simulink model "testing_C_functions5"  (R2020b)
settings: Solver=VariableStepAuto  StartTime=0.0  StopTime=1.5  FixedStep=Ts
undefined symbols (not defined in the file or in its folder): A_frq_step, A_phase_step, DiscIntNeverNeededParam, f_rad, k_phi, ki, kp, N, t_frq_step, t_phase_step, Ts, V_g, var_noise
libraries: simulink x10, bach_library x6
settings Model: Creator=Kasper Laustsen  LastModifiedBy=Kasper Laustsen
settings DataIOCC: ExternalInput=tt1  LoadExternalInput=on
settings SFSimCC: SimCustomHeaderCode=|
  | #include "PLL.h"
  | #include "MAF.h"
settings SFSimCC: SimUserSources=|
  | PLL.c
  | MAF.c

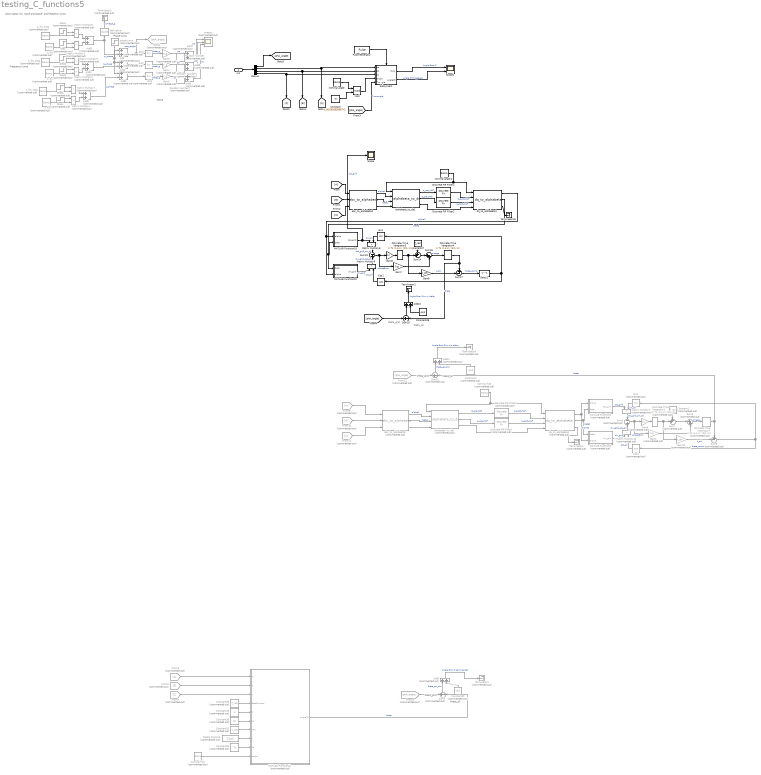
== system testing_C_functions5 ==
  note: Noise
  note: Phase-jump
  note: Input signal incl. noise and phase- and frequency jump
  note: Frequency-jump
  note: theta_pll
  note: theta_grid
  note: theta_pll
  note: theta_grid
  note: theta_pll
  note: theta_grid
  In1 : Inport
  Add{,1..9,11} (11 alike) : Sum  Commented=on
  Add10 : Sum
  Constant : Constant  Value=3.1415926535897*2
  Constant1 : Constant  Commented=on  Value=f_rad
  Constant2 : Constant  Commented=on  Value=-pi/2
  Constant25 : Constant  Commented=on  Value=Ts
  Constant26 : Constant  Commented=on  Value=f_rad
  Constant27 : Constant  Value=f_rad
  Constant28 : Constant  Value=-pi/2
  Constant29 : Constant  Commented=on  Value=ki
  Constant30 : Constant  Commented=on  Value=kp
  Constant31 : Constant  Commented=on  Value=k_phi
  Constant32 : Constant  Commented=on  Value=-pi/2
  Cos1 : Trigonometry  Operator=cos
  Cos2 : Trigonometry  Commented=on  Operator=cos
  Delay2 : Delay  DelayLength=1
  Demux : Demux
  Derivative : Derivative  Commented=on
  Digital Clock12 : DigitalClock  Commented=on  SampleTime=Ts
  Discrete FIR Filter1 : DiscreteFir  Commented=on  Coefficients=[ones(1,round(N)).*1/N]  SampleTime=Ts
  Discrete FIR Filter2 : DiscreteFir  Coefficients=[ones(1,round(N)).*1/N]  SampleTime=Ts
  Discrete FIR Filter3 : DiscreteFir  Commented=on  Coefficients=[ones(1,round(N)).*1/N]  SampleTime=Ts
  Discrete FIR Filter4 : DiscreteFir  Coefficients=[ones(1,round(N)).*1/N]  SampleTime=Ts
  Discrete-Time Integrator1 : DiscreteIntegrator  Commented=on  IntegratorMethod=Integration: Trapezoidal  SampleTime=-1  ICPrevOutput=DiscIntNeverNeededParam  ICPrevScaledInput=DiscIntNeverNeededParam
  Discrete-Time Integrator2 : DiscreteIntegrator  Commented=on  IntegratorMethod=Integration: Trapezoidal  SampleTime=-1  ICPrevOutput=DiscIntNeverNeededParam  ICPrevScaledInput=DiscIntNeverNeededParam
  Discrete-Time Integrator3 : DiscreteIntegrator  IntegratorMethod=Integration: Trapezoidal  SampleTime=-1  ICPrevOutput=DiscIntNeverNeededParam  ICPrevScaledInput=DiscIntNeverNeededParam
  Discrete-Time Integrator4 : DiscreteIntegrator  IntegratorMethod=Integration: Trapezoidal  SampleTime=-1  ICPrevOutput=DiscIntNeverNeededParam  ICPrevScaledInput=DiscIntNeverNeededParam
  From10 : From  Commented=on  GotoTag=B
  From11 : From  Commented=on  GotoTag=C
  From12 : From  Commented=on  GotoTag=phA_angle
  From5 : From  Commented=on
  From6 : From  Commented=on  GotoTag=B
  From7 : From  Commented=on  GotoTag=C
  From8 : From  Commented=on  GotoTag=phA_angle
  From9 : From  Commented=on
  Gain10 : Gain  Commented=on  Gain=k_phi
  Gain2 : Gain  Commented=on  Gain=kp
  Gain3 : Gain  Commented=on  Gain=V_g
  Gain4 : Gain  Commented=on  Gain=V_g
  Gain5 : Gain  Commented=on  Gain=V_g
  Gain6 : Gain  Commented=on  Gain=ki
  Gain7 : Gain  Gain=kp
  Gain8 : Gain  Gain=ki
  Gain9 : Gain  Gain=k_phi
  Goto4 : Goto  Commented=on  GotoTag=phA_angle
  MATLAB Function19 : MATLAB Function  TreatAsAtomicUnit=on
  MATLAB Function2 : MATLAB Function  Commented=on  TreatAsAtomicUnit=on
  MATLAB Function20 : MATLAB Function  TreatAsAtomicUnit=on
  MATLAB Function21 : MATLAB Function  Commented=on  TreatAsAtomicUnit=on
  MATLAB Function3 : MATLAB Function  Commented=on  TreatAsAtomicUnit=on
  Matrix Multiply{1..7,10} (8 alike) : Product  Commented=on
  Matrix Multiply8 : Product
  Matrix Multiply9 : Product
  Mod : Math  Operator=mod  SaturateOnIntegerOverflow=on
  Pulse Generator : DiscretePulseGenerator  PulseType=Time based  Period=Ts  PulseWidth=50
  Random Number : RandomNumber  Commented=on  Variance=var_noise  SampleTime=Ts
  Random Number1 : RandomNumber  Commented=on  Variance=var_noise  Seed=1  SampleTime=Ts
  Random Number2 : RandomNumber  Commented=on  Variance=var_noise  Seed=2  SampleTime=Ts
  Scope : Scope
  Scope1 : Scope  NumInputPorts=2
  Sin1 : Trigonometry
  Sin{2..5} (4 alike) : Trigonometry  Commented=on
  Step : Step  Commented=on  Time=t_frq_step  Before=1  After=0  SampleTime=0
  Step1 : Step  Commented=on  Time=t_frq_step  SampleTime=0
  Step2 : Step  Commented=on  Time=t_frq_step  Before=1  After=0  SampleTime=0
  Step3 : Step  Commented=on  Time=t_frq_step  SampleTime=0
  Step4 : Step  Commented=on  Time=t_frq_step  Before=1  After=0  SampleTime=0
  Step5 : Step  Commented=on  Time=t_frq_step  SampleTime=0
  Subsystem : Subsystem
  Sum10 : Sum  Commented=on  Inputs=+|-
  Sum23 : Sum  Inputs=-|+
  Sum24 : Sum  Inputs=++|
  Sum25 : Sum  Inputs=+|-
  Sum26 : Sum  Inputs=|++
  Sum27 : Sum  Inputs=+-|
  Sum5 : Sum  Commented=on  Inputs=+|-
  Sum6 : Sum  Commented=on  Inputs=-|+
  Sum7 : Sum  Commented=on  Inputs=++|
  Sum8 : Sum  Commented=on  Inputs=|++
  Sum9 : Sum  Commented=on  Inputs=+-|
  Terminator{1,3..5} (4 alike) : Terminator  Commented=on
  Terminator15 : Terminator
  Terminator2 : Terminator
  a_frq : simulink/Sources/Ramp  Commented=on  slope=f_rad  start=0  InitialOutput=0
  a_frq_step : simulink/Sources/Ramp  Commented=on  slope=f_rad*A_frq_step  start=t_frq_step  InitialOutput=t_frq_step*f_rad
  abc_to_alphabeta1 : bach_library/abc_to_alphabeta  SystemSampleTime=-1  VariantActivationTime=update diagram  Latency=0  AutoFrameSizeCalculation=off
  abc_to_alphabeta2 : bach_library/abc_to_alphabeta  Commented=on  SystemSampleTime=-1  VariantActivationTime=update diagram  Latency=0  AutoFrameSizeCalculation=off
  alphabeta_to_dq1 : bach_library/alphabeta_to_dq  SystemSampleTime=-1  VariantActivationTime=update diagram  Latency=0  AutoFrameSizeCalculation=off
  alphabeta_to_dq2 : bach_library/alphabeta_to_dq  Commented=on  SystemSampleTime=-1  VariantActivationTime=update diagram  Latency=0  AutoFrameSizeCalculation=off
  b_frq : simulink/Sources/Ramp  Commented=on  slope=f_rad  start=0  InitialOutput=-pi*2/3
  b_frq_step : simulink/Sources/Ramp  Commented=on  slope=f_rad*A_frq_step  start=t_frq_step  InitialOutput=t_frq_step*f_rad-pi*2/3
  c_frq : simulink/Sources/Ramp  Commented=on  slope=f_rad  start=0  InitialOutput=pi*2/3
  c_frq_step : simulink/Sources/Ramp  Commented=on  slope=f_rad*A_frq_step  start=t_frq_step  InitialOutput=t_frq_step*f_rad+pi*2/3
  dq_to_alphabeta1 : bach_library/dq_to_alphabeta  SystemSampleTime=-1  VariantActivationTime=update diagram  Latency=0  AutoFrameSizeCalculation=off
  dq_to_alphabeta2 : bach_library/dq_to_alphabeta  Commented=on  SystemSampleTime=-1  VariantActivationTime=update diagram  Latency=0  AutoFrameSizeCalculation=off
  "nominal angle " : simulink/Sources/Ramp  slope=f_rad  start=0  InitialOutput=0
  nominal angle 2 : simulink/Sources/Ramp  slope=f_rad  start=0  InitialOutput=0
  nominal frq1 : simulink/Sources/Ramp  Commented=on  slope=f_rad  start=0  InitialOutput=0
  nominal frq3 : simulink/Sources/Ramp  Commented=on  slope=f_rad  start=0  InitialOutput=0
  phase-jump : Step  Commented=on  Time=t_phase_step  After=A_phase_step  SampleTime=0
  phases : Scope  Commented=on  NumInputPorts=3
  wires:
  Matrix Multiply4/1 -> Add5/2
  Matrix Multiply6/1 -> Add3/1
  Step2/1 -> Matrix Multiply2/1
  Matrix Multiply7/1 -> Add5/1
  Step4/1 -> Matrix Multiply4/1
  a_frq_step/1 -> Matrix Multiply6/2
  a_frq/1 -> Matrix Multiply5/2
  Step/1 -> Matrix Multiply5/1
  Sin5/1 -> Gain5/1  "theta_g"
  Gain5/1 -> Add9/1  "pc"
  Step5/1 -> Matrix Multiply7/1
  Matrix Multiply2/1 -> Add4/2
  Add5/1 -> Add2/2  "c_phase"
  c_frq_step/1 -> Matrix Multiply7/2
  b_frq/1 -> Matrix Multiply2/2
  Gain4/1 -> Add8/1  "pb"
  phase-jump/1 -> Add/1, Add2/1, Add1/1
  Add4/1 -> Add1/2  "b_phase"
  Add3/1 -> Add/2, Derivative/1  "a_phase"
  Random Number2/1 -> Add9/2
  b_frq_step/1 -> Matrix Multiply3/2
  Gain3/1 -> Add7/1  "pa"
  Sin4/1 -> Gain4/1  "theta_g"
  Add1/1 -> Sin4/1
  Random Number/1 -> Add7/2
  c_frq/1 -> Matrix Multiply4/2
  Add2/1 -> Sin5/1
  Random Number1/1 -> Add8/2
  Sin3/1 -> Gain3/1  "theta_g"
  Matrix Multiply5/1 -> Add3/2
  Step3/1 -> Matrix Multiply3/1
  Matrix Multiply3/1 -> Add4/1
  Step1/1 -> Matrix Multiply6/1
  Derivative/1 -> Terminator3/1  "omega_g"
  Sum27/1 -> Delay2/1  "theta_comp"
  Sum25/1 -> Add10/1
  alphabeta_to_dq1/3 -> dq_to_alphabeta1/4
  Gain7/1 -> Sum26/2
  Gain8/1 -> Discrete-Time Integrator3/1
  Constant27/1 -> Sum24/1
  dq_to_alphabeta1/3 -> Terminator15/1
  Cos1/1 -> Matrix Multiply9/2  "cos_pll"
  MATLAB Function20/1(sin_grid) -> Matrix Multiply9/1  "sin_grid"
  Gain9/1 -> Sum27/2  "k_phi"
  Add/1 -> Goto4/1, Sin3/1  "pha_angle"
  abc_to_alphabeta1/3 -> alphabeta_to_dq1/4
  abc_to_alphabeta1/1 -> alphabeta_to_dq1/2  "alpha1"
  Discrete FIR Filter4/1 -> dq_to_alphabeta1/2  "d_post_MAF"
  abc_to_alphabeta1/2 -> alphabeta_to_dq1/3  "beta1"
  dq_to_alphabeta1/2 -> MATLAB Function20/1(beta), MATLAB Function19/2(beta)  "beta2"
  nominal angle 2/1 -> dq_to_alphabeta1/1, alphabeta_to_dq1/1
  Add8/1 -> phases/2  "pb"
  Sin1/1 -> Matrix Multiply8/2  "sin_pll"
  Discrete-Time Integrator4/1 -> Sum27/1, Sum25/2  "theta"
  Sum24/1 -> Sum26/1
  alphabeta_to_dq1/1 -> Discrete FIR Filter4/1  "d_pre_MAF"
  Sum26/1 -> Discrete-Time Integrator4/1  "omega"
  Discrete FIR Filter2/1 -> dq_to_alphabeta1/3  "q_post_MAF"
  Add10/1 -> Terminator2/1  "Angle Error Sim w. delay"
  Matrix Multiply9/1 -> Sum23/2  "sin_grid_cos_pll"
  alphabeta_to_dq1/2 -> Discrete FIR Filter2/1  "q_pre_MAF"
  dq_to_alphabeta1/1 -> MATLAB Function20/2(alpha), MATLAB Function19/1(alpha)  "alpha2"
  Add9/1 -> phases/3  "pc"
  Matrix Multiply8/1 -> Sum23/1  "cos_grid_sin_pll"
  Constant28/1 -> Add10/2
  Discrete-Time Integrator3/1 -> Sum24/2, Gain9/1
  Add7/1 -> phases/1  "pa"
  MATLAB Function19/1(cos_grid) -> Scope/1, Matrix Multiply8/1  "cos_grid"
  Sum23/1 -> Gain8/1, Gain7/1  "phaseError"
  Delay2/1 -> Sin1/1, Cos1/1
  [phA_angle] -> Sum25/1
  [C] -> abc_to_alphabeta1/3
  [B] -> abc_to_alphabeta1/2
  [A] -> abc_to_alphabeta1/1
  Constant25/1 -> MATLAB Function21/9(Ts)
  Constant30/1 -> MATLAB Function21/6(kp)
  Constant31/1 -> MATLAB Function21/7(kPhi)
  Constant29/1 -> MATLAB Function21/5(ki)
  Constant26/1 -> MATLAB Function21/4(feedForward)
  Digital Clock12/1 -> MATLAB Function21/8(t)
  From7/1 -> MATLAB Function21/3(c)
  From6/1 -> MATLAB Function21/2(b)
  From5/1 -> MATLAB Function21/1(a)
  nominal frq1/1 -> MATLAB Function21/10(angle)
  From8/1 -> Sum5/1
  Add6/1 -> Terminator1/1  "Angle Error C sammensat"
  Sum5/1 -> Add6/1  "theta_err_sim"
  MATLAB Function21/1(anglePll) -> Sum5/2  "theta"
  Constant32/1 -> Add6/2
  Pulse Generator/1 -> Subsystem/Trigger
  [phA_angle] -> Subsystem/5(True angle)  "True angle"
  Subsystem/1(Out1) -> Scope1/1  "Angle Error C"
  Subsystem/2(anglePll) -> Scope1/2  "Angle Pll triggered"
  Discrete FIR Filter3/1 -> dq_to_alphabeta2/2  "d_post_MAF"
  From11/1 -> abc_to_alphabeta2/3
  Discrete FIR Filter1/1 -> dq_to_alphabeta2/3  "q_post_MAF"
  Gain10/1 -> Sum9/2  "k_phi"
  Sum6/1 -> Gain6/1, Gain2/1  "phaseError"
  MATLAB Function2/1(cos_grid) -> Matrix Multiply1/1  "cos_grid"
  Sum7/1 -> Sum8/1
  Matrix Multiply1/1 -> Sum6/1  "cos_grid_sin_pll"
  Sin2/1 -> Matrix Multiply1/2  "sin_pll"
  abc_to_alphabeta2/1 -> alphabeta_to_dq2/2  "alpha1"
  dq_to_alphabeta2/1 -> MATLAB Function2/1(alpha), MATLAB Function3/2(alpha)  "alpha2"
  dq_to_alphabeta2/2 -> MATLAB Function3/1(beta), MATLAB Function2/2(beta)  "beta2"
  alphabeta_to_dq2/1 -> Discrete FIR Filter3/1  "d_pre_MAF"
  MATLAB Function3/1(sin_grid) -> Matrix Multiply10/1  "sin_grid"
  Sum9/1 -> Sin2/1, Cos2/1  "theta_comp"
  dq_to_alphabeta2/3 -> Terminator4/1
  Gain6/1 -> Discrete-Time Integrator1/1
  Gain2/1 -> Sum8/2
  Matrix Multiply10/1 -> Sum6/2  "sin_grid_cos_pll"
  Discrete-Time Integrator2/1 -> Sum10/2, Sum9/1  "theta"
  nominal frq3/1 -> dq_to_alphabeta2/1, alphabeta_to_dq2/1
  Cos2/1 -> Matrix Multiply10/2  "cos_pll"
  abc_to_alphabeta2/2 -> alphabeta_to_dq2/3  "beta1"
  From9/1 -> abc_to_alphabeta2/1
  alphabeta_to_dq2/3 -> dq_to_alphabeta2/4
  Sum8/1 -> Discrete-Time Integrator2/1  "omega"
  From10/1 -> abc_to_alphabeta2/2
  Constant1/1 -> Sum7/1
  abc_to_alphabeta2/3 -> alphabeta_to_dq2/4
  Discrete-Time Integrator1/1 -> Sum7/2, Gain10/1
  alphabeta_to_dq2/2 -> Discrete FIR Filter1/1  "q_pre_MAF"
  Constant2/1 -> Add11/2
  Add11/1 -> Terminator5/1  "Angle Error Sim w/o delay"
  Sum10/1 -> Add11/1  "theta_err_sim"
  From12/1 -> Sum10/1
  In1/1 -> Demux/1
  Demux/2 -> [A], Subsystem/1(pa)
  Demux/3 -> [B], Subsystem/2(pb)
  Demux/4 -> Subsystem/3(pc), [C]
  Demux/1 -> [phA_angle]
  "nominal angle "/1 -> Mod/1
  Mod/1 -> Subsystem/4("angle ")
  Constant/1 -> Mod/2

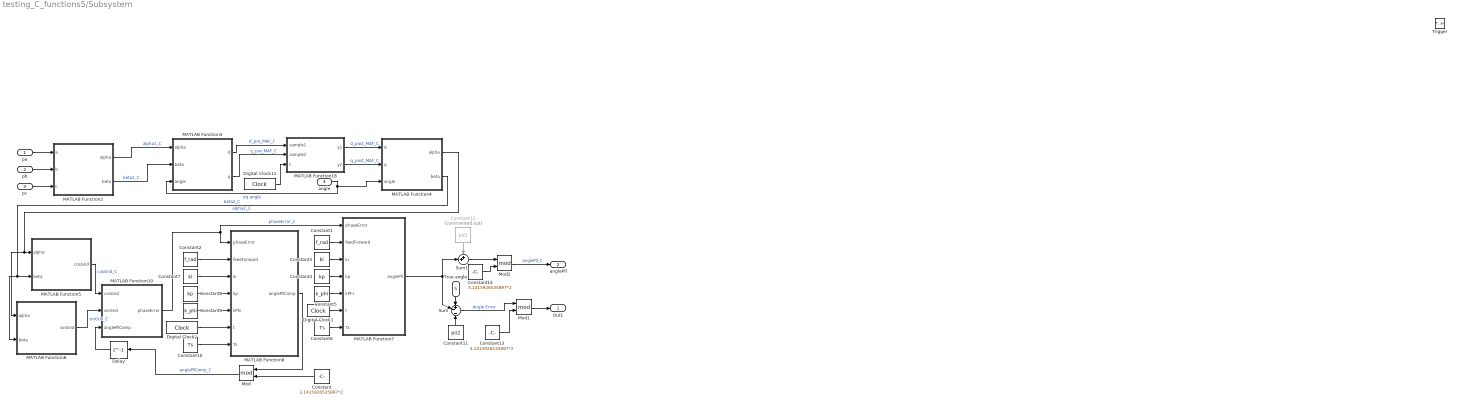
== system testing_C_functions5/Subsystem ==
  pa : Inport
  pb : Inport  Port=2
  pc : Inport  Port=3
  "angle " : Inport  Port=4
  True angle : Inport  Port=5
  Trigger : TriggerPort  VariantControl=Variant  PortDimensions=1
  Constant : Constant  Value=3.1415926535897*2
  Constant1 : Constant  Value=f_rad
  Constant10 : Constant  Value=Ts
  Constant11 : Constant  Value=pi/2
  Constant12 : Constant  Commented=on  Value=pi/2
  Constant13 : Constant  Value=3.1415926535897*2
  Constant14 : Constant  Value=3.1415926535897*2
  Constant2 : Constant  Value=f_rad
  Constant3 : Constant  Value=ki
  Constant4 : Constant  Value=kp
  Constant5 : Constant  Value=k_phi
  Constant6 : Constant  Value=Ts
  Constant7 : Constant  Value=ki
  Constant8 : Constant  Value=kp
  Constant9 : Constant  Value=k_phi
  Delay : Delay  DelayLength=1
  Digital Clock1 : DigitalClock  SampleTime=-1
  Digital Clock11 : DigitalClock  SampleTime=-1
  Digital Clock2 : DigitalClock  SampleTime=-1
  MATLAB Function10 : MATLAB Function  TreatAsAtomicUnit=on
  MATLAB Function18 : MATLAB Function  TreatAsAtomicUnit=on
  MATLAB Function2 : MATLAB Function  TreatAsAtomicUnit=on
  MATLAB Function3 : MATLAB Function  TreatAsAtomicUnit=on
  MATLAB Function4 : MATLAB Function  TreatAsAtomicUnit=on
  MATLAB Function5 : MATLAB Function  TreatAsAtomicUnit=on
  MATLAB Function6 : MATLAB Function  TreatAsAtomicUnit=on
  MATLAB Function7 : MATLAB Function  TreatAsAtomicUnit=on
  MATLAB Function8 : MATLAB Function  TreatAsAtomicUnit=on
  Mod : Math  Operator=mod  SaturateOnIntegerOverflow=on
  Mod1 : Math  Operator=mod  SaturateOnIntegerOverflow=on
  Mod2 : Math  Operator=mod  SaturateOnIntegerOverflow=on
  Sum : Sum  Inputs=+-|-
  Sum1 : Sum  Inputs=++|
  Out1 : Outport
  anglePll : Outport  Port=2
  wires:
  MATLAB Function5/1(cosGrid) -> MATLAB Function10/1(cosGrid)  "cosGrid_C"
  MATLAB Function2/1(alpha) -> MATLAB Function3/1(alpha)  "alpha1_C"
  MATLAB Function7/1(anglePll) -> Sum1/2, Sum/2
  Constant10/1 -> MATLAB Function8/7(Ts)
  Delay/1 -> MATLAB Function10/3(anglePllComp)
  MATLAB Function6/1(sinGrid) -> MATLAB Function10/2(sinGrid)  "sinGrid_C"
  MATLAB Function4/1(alpha) -> MATLAB Function6/1(alpha), MATLAB Function5/1(alpha)  "alpha2_C"
  True angle/1 -> Sum/1
  Constant7/1 -> MATLAB Function8/3(ki)
  Digital Clock1/1 -> MATLAB Function7/6(t)
  MATLAB Function18/2(y2) -> MATLAB Function4/2(q)  "q_post_MAF_C"
  MATLAB Function4/2(beta) -> MATLAB Function6/2(beta), MATLAB Function5/2(beta)  "beta2_C"
  Digital Clock2/1 -> MATLAB Function8/6(t)
  Digital Clock11/1 -> MATLAB Function18/3(t)
  MATLAB Function2/2(beta) -> MATLAB Function3/2(beta)  "beta1_C"
  Constant5/1 -> MATLAB Function7/5(kPhi)
  Constant3/1 -> MATLAB Function7/3(ki)
  Constant8/1 -> MATLAB Function8/4(kp)
  Constant1/1 -> MATLAB Function7/2(feedForward)
  Constant2/1 -> MATLAB Function8/2(feedForward)
  pa/1 -> MATLAB Function2/1(a)
  MATLAB Function10/1(phaseError) -> MATLAB Function7/1(phaseError), MATLAB Function8/1(phaseError)  "phaseError_C"
  MATLAB Function18/1(y1) -> MATLAB Function4/1(d)  "d_post_MAF_C"
  MATLAB Function3/2(q) -> MATLAB Function18/2(sample2)  "q_pre_MAF_C"
  Constant9/1 -> MATLAB Function8/5(kPhi)
  Constant4/1 -> MATLAB Function7/4(kp)
  MATLAB Function3/1(d) -> MATLAB Function18/1(sample1)  "d_pre_MAF_C"
  "angle "/1 -> MATLAB Function4/3(angle), MATLAB Function3/3(angle)  "dq angle"
  Constant11/1 -> Sum/3
  Constant6/1 -> MATLAB Function7/7(Ts)
  MATLAB Function8/1(anglePllComp) -> Mod/1
  Sum/1 -> Mod1/1  "Angle Error"
  pc/1 -> MATLAB Function2/3(c)
  pb/1 -> MATLAB Function2/2(b)
  Constant12/1 -> Sum1/1
  Sum1/1 -> Mod2/1
  Constant/1 -> Mod/2
  Mod/1 -> Delay/1  "anglePllComp_C"
  Constant13/1 -> Mod1/2
  Mod1/1 -> Out1/1
  Mod2/1 -> anglePll/1  "anglePll_C"
  Constant14/1 -> Mod2/2

== matlab function testing_C_functions5/Subsystem/MATLAB Function18 ==
  data: sample1 input; sample2 input; y1 output; t input; y2 output
function [y1, y2] = calling_moving_avg(sample1, sample2, t)
% coder.updateBuildInfo('addSourceFiles','moving_avg.c');
% coder.cinclude('moving_avg.h');

coder.updateBuildInfo('addSourceFiles','MAF.c');
coder.cinclude('MAF.h');

y1 = 0.0;
y2 = 0.0;
% y = coder.ceval('moving_avg',u,t);
% y1 = coder.ceval('maf1',len, sample1, t);
% y2 = coder.ceval('maf2',len, sample2, t);
y1 = coder.ceval('maf1', sample1, t); %explicit def of length removed
y2 = coder.ceval('maf2', sample2, t); %explicit def of length removed

== matlab function testing_C_functions5/MATLAB Function21 ==
  data: a input; b input; c input; anglePll output; feedForward input; ki input; kp input; kPhi input; t input; Ts input; angle input
function anglePll  = calling_pll(a, b, c, feedForward, ki, kp, kPhi, t, Ts, angle)
% coder.updateBuildInfo('addSourceFiles','abc_to_alphabeta.c');
% coder.cinclude('abc_to_alphabeta.h');
coder.updateBuildInfo('addSourceFiles','PLL.c');
coder.cinclude('PLL.h');

anglePll = 0.0;

anglePll = coder.ceval('pll', a, b, c, feedForward, ki, kp, kPhi, t, Ts, angle);

== matlab function testing_C_functions5/MATLAB Function19 ==
  data: alpha input; cos_grid output; beta input
function cos_grid = cos_grid(alpha, beta)

cos_grid = alpha/sqrt(alpha^2+beta^2);

== matlab function testing_C_functions5/MATLAB Function20 ==
  data: beta input; alpha input; sin_grid output
function sin_grid = sin_grid(beta, alpha)

sin_grid = beta/sqrt(alpha^2+beta^2);

== matlab function testing_C_functions5/MATLAB Function3 ==
  data: beta input; alpha input; sin_grid output
function sin_grid = sin_grid(beta, alpha)

sin_grid = beta/sqrt(alpha^2+beta^2);

== matlab function testing_C_functions5/Subsystem/MATLAB Function2 ==
  data: a input; alpha output; b input; c input; beta output
function [alpha,beta] = calling_abc_to_alphabeta(a,b,c)
% coder.updateBuildInfo('addSourceFiles','abc_to_alphabeta.c');
% coder.cinclude('abc_to_alphabeta.h');
coder.updateBuildInfo('addSourceFiles','PLL.c');
coder.cinclude('PLL.h');


alpha = 0.0;
beta = 0.0;

alpha = coder.ceval('abc_to_alpha',a,b,c);
beta = coder.ceval('abc_to_beta',a,b,c);

== matlab function testing_C_functions5/Subsystem/MATLAB Function3 ==
  data: alpha input; d output; beta input; angle input; q output
function [d, q] = calling_alphabeta_to_dq(alpha, beta, angle)
% coder.updateBuildInfo('addSourceFiles','abc_to_alphabeta.c');
% coder.cinclude('abc_to_alphabeta.h');
coder.updateBuildInfo('addSourceFiles','PLL.c');
coder.cinclude('PLL.h');


d = 0.0;
q = 0.0;

d = coder.ceval('alphabeta_to_d',alpha, beta, angle);
q = coder.ceval('alphabeta_to_q',alpha, beta, angle);

== matlab function testing_C_functions5/Subsystem/MATLAB Function4 ==
  data: d input; alpha output; q input; angle input; beta output
function [alpha, beta] = calling_dq_to_alphabeta(d, q, angle)
% coder.updateBuildInfo('addSourceFiles','abc_to_alphabeta.c');
% coder.cinclude('abc_to_alphabeta.h');
coder.updateBuildInfo('addSourceFiles','PLL.c');
coder.cinclude('PLL.h');


alpha = 0.0;
beta = 0.0;

alpha = coder.ceval('dq_to_alpha', d, q, angle);
beta = coder.ceval('dq_to_beta', d, q, angle);

== matlab function testing_C_functions5/Subsystem/MATLAB Function5 ==
  data: alpha input; cosGrid output; beta input
function cosGrid  = calling_cos_grid(alpha, beta)
% coder.updateBuildInfo('addSourceFiles','abc_to_alphabeta.c');
% coder.cinclude('abc_to_alphabeta.h');
coder.updateBuildInfo('addSourceFiles','PLL.c');
coder.cinclude('PLL.h');

cosGrid = 0.0;

cosGrid = coder.ceval('cos_grid', alpha, beta);

== matlab function testing_C_functions5/Subsystem/MATLAB Function6 ==
  data: alpha input; sinGrid output; beta input
function sinGrid  = calling_sin_grid(alpha, beta)
% coder.updateBuildInfo('addSourceFiles','abc_to_alphabeta.c');
% coder.cinclude('abc_to_alphabeta.h');
coder.updateBuildInfo('addSourceFiles','PLL.c');
coder.cinclude('PLL.h');

sinGrid = 0.0;

sinGrid = coder.ceval('sin_grid', alpha, beta);

== matlab function testing_C_functions5/Subsystem/MATLAB Function7 ==
  data: phaseError input; anglePll output; feedForward input; ki input; kp input; kPhi input; t input; Ts input
function anglePll  = calling_pi_regulator(phaseError, feedForward, ki, kp, kPhi, t, Ts)
% coder.updateBuildInfo('addSourceFiles','abc_to_alphabeta.c');
% coder.cinclude('abc_to_alphabeta.h');
coder.updateBuildInfo('addSourceFiles','PLL.c');
coder.cinclude('PLL.h');

anglePll = 0.0;

anglePll = coder.ceval('pi_regulator', phaseError, feedForward, ki, kp, kPhi, t, Ts);

== matlab function testing_C_functions5/Subsystem/MATLAB Function8 ==
  data: phaseError input; anglePllComp output; feedForward input; ki input; kp input; kPhi input; t input; Ts input
function anglePllComp  = calling_pi_regulator_comp(phaseError, feedForward, ki, kp, kPhi, t, Ts)
% coder.updateBuildInfo('addSourceFiles','abc_to_alphabeta.c');
% coder.cinclude('abc_to_alphabeta.h');
coder.updateBuildInfo('addSourceFiles','PLL.c');
coder.cinclude('PLL.h');

anglePllComp = 0.0;

anglePllComp = coder.ceval('pi_regulator_comp', phaseError, feedForward, ki, kp, kPhi, t, Ts);

== matlab function testing_C_functions5/MATLAB Function2 ==
  data: alpha input; cos_grid output; beta input
function cos_grid = cos_grid(alpha, beta)

cos_grid = alpha/sqrt(alpha^2+beta^2);

== matlab function testing_C_functions5/Subsystem/MATLAB Function10 ==
  data: cosGrid input; phaseError output; sinGrid input; anglePllComp input
function phaseError  = calling_phase_detector(cosGrid, sinGrid, anglePllComp)
% coder.updateBuildInfo('addSourceFiles','abc_to_alphabeta.c');
% coder.cinclude('abc_to_alphabeta.h');
coder.updateBuildInfo('addSourceFiles','PLL.c');
coder.cinclude('PLL.h');

phaseError = 0.0;

phaseError = coder.ceval('phase_detector', cosGrid, sinGrid, anglePllComp);
